simulink model "Det_Inv_Polynom_Quad__MATRICES"  (R2018b)
settings: Solver=VariableStepAuto  StartTime=0.0  StopTime=10.0  RelTol=1e-3
values from neighbouring files (symbols this model uses):
  A = input('Enter a given Matrix: ')    [Chol_decomposition.m]    (also in LA_ex2.m = magic(13); LA_ex3.m = randi([-100,100],100); LA_ex4.m = [.072, 0, -1; 0, .12, -1; 1 1 0]; LU_decomposition.m = input('Enter rectangular matrix: '))
  B = randi([-169,169], 13,1)    [LA_ex2.m]    (also in LA_ex3.m = randi([-100, 100], 100, 1); LA_ex4.m = [-12; -9; Bk(ii)])
undefined symbols (not defined in the file or in its folder): A1, B1
libraries: dspmtrx3 x3, dspsolvers x3, dspinverses x2, sharedutil x2, aerolibutil x1
settings Model: Creator=sulaymon.eshkabilov  LastModifiedBy=sulaymon.eshkabilov

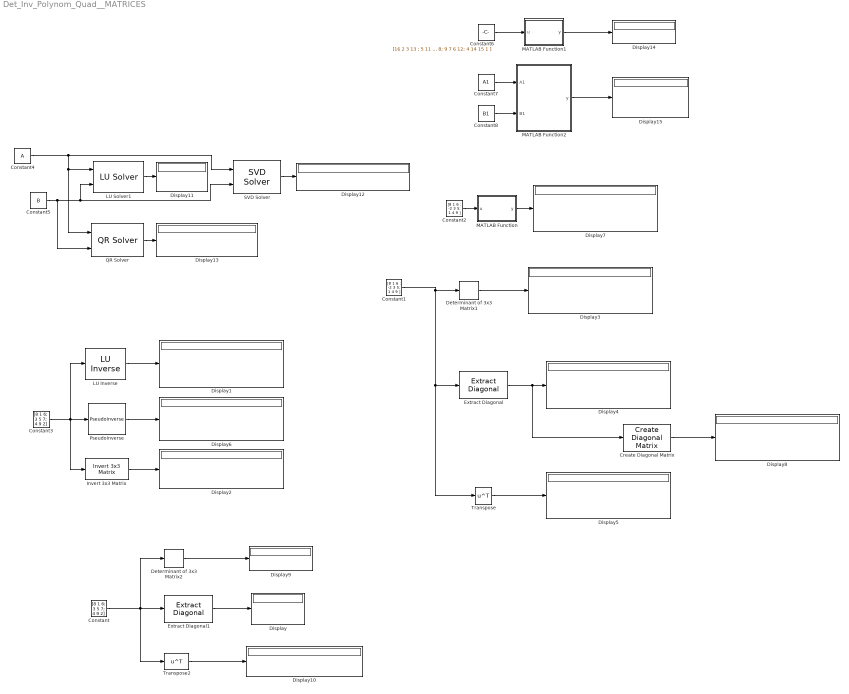
== system Det_Inv_Polynom_Quad__MATRICES ==
  " LU Inverse" : dspinverses/ LU Inverse
      settings: SourceProductName=DSP System Toolbox
  Constant : Constant  Value=[8 1 6; 3 5 7; 4 9 2]
  Constant1 : Constant  Value=[8 1 6 ; -2 3 5; 1 4 9 ]
  Constant2 : Constant  Value=[8 1 6 ; -2 3 5; 1 4 9 ]
  Constant3 : Constant  Value=[8 1 6; 3 5 7; 4 9 2]
  Constant4 : Constant  Value=A
  Constant5 : Constant  Value=B
  Constant6 : Constant  Value=[16 2 3 13 ; 5 11 10 8; 9 7 6 12; 4 14 15 1 ]
  Constant7 : Constant  Value=A1
  Constant8 : Constant  Value=B1
  Create Diagonal Matrix : dspmtrx3/Create Diagonal Matrix
      settings: SourceProductName=DSP System Toolbox  SourceProductBaseCode=DS
  Determinant of 3x3 Matrix1 : sharedutil/Determinant of 3x3 Matrix  aMode=aMode
      settings: SourceProductName=Aerospace Blockset  SourceProductBaseCode=AE
  Determinant of 3x3 Matrix2 : sharedutil/Determinant of 3x3 Matrix  aMode=aMode
      settings: SourceProductName=Aerospace Blockset  SourceProductBaseCode=AE
  Display{,1..15} (16 alike) : Display
      Display11 settings: Format=hex (Stored Integer)  Decimation=16
      Display12 settings: Format=short_e  Decimation=16
      Display13 settings: Decimation=16
      Display15 settings: Format=long_e
  Extract Diagonal : dspmtrx3/Extract Diagonal
      settings: SourceProductName=DSP System Toolbox  SourceProductBaseCode=DS
  Extract Diagonal1 : dspmtrx3/Extract Diagonal
      settings: SourceProductName=DSP System Toolbox  SourceProductBaseCode=DS
  Invert 3x3 Matrix : aerolibutil/Invert  3x3 Matrix
  LU Solver1 : dspsolvers/LU Solver
      settings: SourceProductName=DSP System Toolbox  SourceProductBaseCode=DS
  MATLAB Function : MATLAB Function  TreatAsAtomicUnit=on
  MATLAB Function1 : MATLAB Function  TreatAsAtomicUnit=on
  MATLAB Function2 : MATLAB Function  TreatAsAtomicUnit=on
  Pseudoinverse : dspinverses/Pseudoinverse  wanterr=off  SimulateUsing=Interpreted execution
      settings: SourceProductName=DSP System Toolbox  SourceProductBaseCode=DS
  QR Solver : dspsolvers/QR Solver
      settings: SourceProductName=DSP System Toolbox  SourceProductBaseCode=DS
  SVD Solver : dspsolvers/SVD Solver  wanterr=off
      settings: SourceProductName=DSP System Toolbox  SourceProductBaseCode=DS
  Transpose : Math  Operator=transpose  SaturateOnIntegerOverflow=on
  Transpose2 : Math  Operator=transpose  RndMeth=Zero  SaturateOnIntegerOverflow=on
  wires:
  Constant3/1 -> Invert 3x3 Matrix/1, " LU Inverse"/1, Pseudoinverse/1
  Pseudoinverse/1 -> Display6/1
  " LU Inverse"/1 -> Display1/1
  Invert 3x3 Matrix/1 -> Display2/1
  Constant1/1 -> Transpose/1, Extract Diagonal/1, Determinant of 3x3 Matrix1/1
  Determinant of 3x3 Matrix1/1 -> Display3/1
  Extract Diagonal/1 -> Create Diagonal Matrix/1, Display4/1
  Transpose/1 -> Display5/1
  Constant2/1 -> MATLAB Function/1(u)
  MATLAB Function/1(y) -> Display7/1
  Create Diagonal Matrix/1 -> Display8/1
  Constant/1 -> Transpose2/1, Determinant of 3x3 Matrix2/1, Extract Diagonal1/1
  Extract Diagonal1/1 -> Display/1
  Determinant of 3x3 Matrix2/1 -> Display9/1
  Transpose2/1 -> Display10/1
  Constant5/1 -> QR Solver/2, LU Solver1/2, SVD Solver/2
  Constant4/1 -> SVD Solver/1, LU Solver1/1, QR Solver/1
  QR Solver/1 -> Display13/1
  SVD Solver/1 -> Display12/1
  LU Solver1/1 -> Display11/1
  Constant7/1 -> MATLAB Function2/1(A1)
  Constant8/1 -> MATLAB Function2/2(B1)
  MATLAB Function2/1(y) -> Display15/1
  Constant6/1 -> MATLAB Function1/1(u)
  MATLAB Function1/1(y) -> Display14/1

== matlab function Det_Inv_Polynom_Quad__MATRICES/MATLAB Function1 ==
  data: u input; y output
function y = fcn(u)
y = det(u);

== matlab function Det_Inv_Polynom_Quad__MATRICES/MATLAB Function ==
  data: u input; y output
function y = fcn(u)
y = det(u);

== matlab function Det_Inv_Polynom_Quad__MATRICES/MATLAB Function2 ==
  data: A1 input; y output; B1 input
function y = fcn(A1, B1)
y = linsolve(A1, B1);
